simulink model "simulink_openloop_modelb_control101"  (R2023a)
settings: Solver=ode45  StartTime=0.0  StopTime=t_stop  RelTol=1e-3  EnableMultiTasking=on
values from neighbouring files (symbols this model uses):
  B = 500    [simulink_openloop_model_control101_script.m]    (also in simulink_openloop_modelb_control101_script.m; simulink_openloop_modelc_control101_script.m; simulink_openloop_modeld_control101_script.m)
  C = 6000    [simulink_openloop_model_control101_script.m]    (also in simulink_openloop_modelb_control101_script.m; simulink_openloop_modelc_control101_script.m = 2000; simulink_openloop_modeld_control101_script.m = 1000)
  M = 1000    [simulink_openloop_model_control101_script.m]    (also in simulink_openloop_modelb_control101_script.m; simulink_openloop_modelc_control101_script.m; simulink_openloop_modeld_control101_script.m)
  Mg = M*10    (= 10000)    [simulink_openloop_modelb_control101_script.m]
settings Model: Creator=uos  LastModifiedBy=Anthony Rossiter
settings SolverCC: AlgebraicLoopSolver=TrustRegion
settings DataIOCC: LimitDataPoints=on  SaveFormat=Array  SignalLoggingSaveFormat=ModelDataLogs  ReturnWorkspaceOutputs=off
settings OptimizationCC: BooleanDataType=off  ExpressionDepthLimit=2147483647  LifeSpan=inf
settings DebuggingCC: SaveWithParameterizedLinksMsg=none  UnderspecifiedInitializationDetection=Classic  MergeDetectMultiDrivingBlocksExec=none  SignalResolutionControl=TryResolveAllWithWarning  MultiTaskDSMMsg=warning  MultiTaskCondExecSysMsg=none  FcnCallInpInsideContextMsg=warning  UnconnectedInputMsg=warning  UnconnectedOutputMsg=warning  UnconnectedLineMsg=warning  StateNameClashWarn=warning  SFUnexpectedBacktrackingDiag=warning  SFNoUnconditionalDefaultTransitionDiag=warning  SFExecutionAtInitializationDiag=none  ArithmeticOperatorsInVariantConditions=warning
settings HardwareCC: ProdBitPerPointer=32  ProdBitPerSizeT=32  ProdBitPerPtrDiffT=32  ProdLargestAtomicFloat=None  ProdIntDivRoundTo=Undefined  ProdEndianess=Unspecified  ProdWordSize=32  ProdHWDeviceType=32-bit Generic  TargetUnknown=on
settings ModelReferenceCC: EnableRefExpFcnMdlSchedulingChecks=on  PropagateSignalLabelsOutOfModel=off
settings SFSimCC: SimUseLocalCustomCode=off  CustomCodeUndefinedFunction=UseInterfaceOnly
settings RTWCC: RTWUseLocalCustomCode=off  DLArmComputeVersion=19.05
settings CodeAppCC: StateflowObjectComments=on
settings GRTTargetCC: TargetLangStandard=C89/C90 (ANSI)  CombineOutputUpdateFcns=off  GRTInterface=on
settings ConfigComp: CovMetricSettings=dw  CovSaveCumulativeToWorkspaceVar=on  CovSaveSingleToWorkspaceVar=on  CovExternalEMLEnable=off

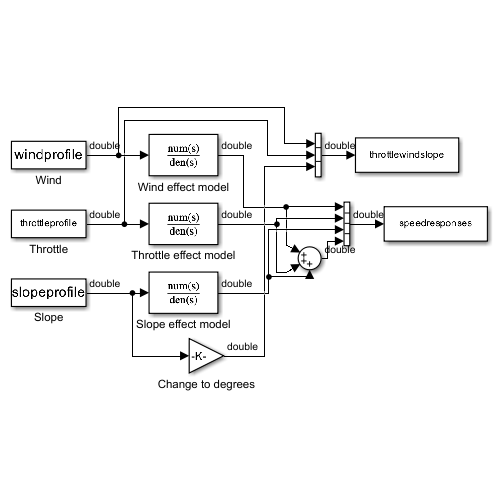
[thumbnail: Simulink's stored preview of the top-level diagram]
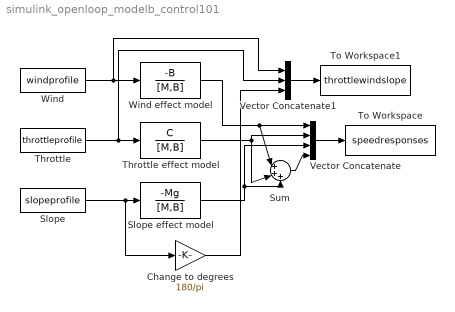
== system simulink_openloop_modelb_control101 ==
  Change to degrees : Gain  Gain=180/pi
  Slope : FromWorkspace  VariableName=slopeprofile  Interpolate=off  ZeroCross=off  OutputAfterFinalValue=Holding final value
  Slope effect model : TransferFcn  Numerator=-Mg  Denominator=[M,B]
  Sum : Sum  Inputs=|+++
  Throttle : FromWorkspace  VariableName=throttleprofile  Interpolate=off  ZeroCross=off  OutputAfterFinalValue=Holding final value
  Throttle effect model : TransferFcn  Numerator=C  Denominator=[M,B]
  To Workspace : ToWorkspace  VariableName=speedresponses  SaveFormat=Structure With Time  SampleTime=-1
  To Workspace1 : ToWorkspace  VariableName=throttlewindslope  SaveFormat=Structure With Time  SampleTime=-1
  Vector Concatenate : Concatenate  NumInputs=4
  Vector Concatenate1 : Concatenate  NumInputs=3
  Wind : FromWorkspace  VariableName=windprofile  Interpolate=off  ZeroCross=off  OutputAfterFinalValue=Holding final value
  Wind effect model : TransferFcn  Numerator=-B  Denominator=[M,B]
  wires:
  Throttle/1 -> Vector Concatenate1/2, Throttle effect model/1
  Wind/1 -> Vector Concatenate1/1, Wind effect model/1
  Wind effect model/1 -> Sum/1, Vector Concatenate/1
  Slope effect model/1 -> Sum/3, Vector Concatenate/3
  Vector Concatenate/1 -> To Workspace/1
  Vector Concatenate1/1 -> To Workspace1/1
  Sum/1 -> Vector Concatenate/4
  Throttle effect model/1 -> Vector Concatenate/2, Sum/2
  Slope/1 -> Change to degrees/1, Slope effect model/1
  Change to degrees/1 -> Vector Concatenate1/3
